simulink model "OdeSimSpring2"  (R2013a)
settings: Solver=ode15s  StartTime=0.0  StopTime=T  MaxStep=1e-3  RelTol=1e-3
InitFcn:
  | m=.015;
  | K=1000;
  | L0=.08;
  | f=1;
  | T=1/f;
  | L0_Ode=.1;
  | D_L0_Ode=.01;
  | R=.016;
  | 
  | % Constant Velocity
  | a1=(3/2*pi)/T;
  | 
  | % constant acceleration
  | a2=2*(3/2*pi)/((T^2));
  | 
  | % sin
  | a3=-(3/4*pi);
  | b3=pi/T;
  | c3=pi/2;
  | d3=-a3;
libraries: simulink x1
settings Model: Creator=root  LastModifiedBy=root

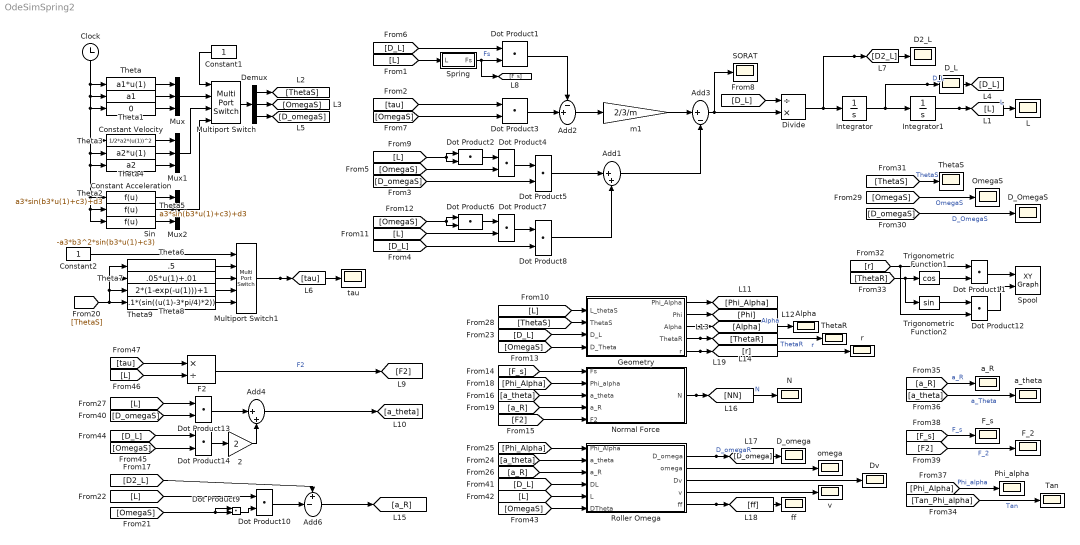
== system OdeSimSpring2 ==
  2 : Gain  Gain=2
  Add1 : Sum  Inputs=|++
  Add2 : Sum  Inputs=-+|
  Add3 : Sum  Inputs=|+-
  Add4 : Sum  Inputs=|++
  Add6 : Sum  Inputs=+-|
  Alpha : Scope
  Clock : Clock
  Constant Acceleration : Fcn  Expr=a2
  Constant Velocity : Fcn  Expr=0
  Constant1 : Constant
  Constant2 : Constant
  D2_L : Scope
      settings: SaveName=ScopeData21
  D_L : Scope
      settings: SaveName=ScopeData22
  D_OmegaS : Scope
      settings: SaveName=ScopeData16
  D_omega : Scope
      settings: TimeRange=1  YMin=-99.79943282286136  YMax=104.2652110780353
  Demux : Demux  Outputs=3
  Divide : Product  Inputs=/*
  Dot Product{1..14} (14 alike) : DotProduct  InputSameDT=on  OutDataTypeStr=Inherit: Inherit via internal rule
  Dv : Scope
      settings: TimeRange=1  YMin=-1.967332415830284  YMax=2.10455506696653  SaveName=ScopeData2
  F2 : Product  Inputs=*/
  F_2 : Scope
      settings: SaveName=ScopeData3
  F_s : Scope
      settings: SaveName=ScopeData4
  Geometry : Subsystem
  Integrator : Integrator  InitialCondition=D_L0_Ode
  Integrator1 : Integrator  InitialCondition=L0_Ode
  L : Scope
      settings: SaveName=ScopeData23
  Multiport Switch : MultiPortSwitch
  Multiport Switch1 : MultiPortSwitch  Inputs=4
  Mux : Mux  Inputs=3
  Mux1 : Mux  Inputs=3
  Mux2 : Mux  Inputs=3
  N : Scope
      settings: SaveName=ScopeData5
  Normal Force : Subsystem
  OmegaS : Scope
      settings: SaveName=ScopeData18
  Phi_alpha : Scope
      settings: SaveName=ScopeData8
  Roller Omega : Subsystem
  SORAT : Scope
      settings: SaveName=ScopeData15
  Sin : Fcn  Expr=-a3*b3^2*sin(b3*u(1)+c3)
  Spool : simulink/Sinks/XY Graph  xmin=-.3  xmax=.3  ymin=-.3  ymax=.3  st=-1
  Spring : Subsystem
  Tan : Scope
      settings: SaveName=ScopeData9
  Theta : Fcn  Expr=a1*u(1)
  Theta1 : Fcn  Expr=a1
  Theta2 : Fcn  Expr=a3*sin(b3*u(1)+c3)+d3
  Theta3 : Fcn  Expr=1/2*a2*(u(1))^2
  Theta4 : Fcn  Expr=a2*u(1)
  Theta5 : Fcn  Expr=a3*sin(b3*u(1)+c3)+d3
  Theta6 : Fcn  Expr=.5
  Theta7 : Fcn  Expr=.05*u(1)+.01
  Theta8 : Fcn  Expr=2*(1-exp(-u(1)))+1
  Theta9 : Fcn  Expr=.1*(sin((u(1)-3*pi/4)*2))
  ThetaR : Scope
      settings: SaveName=ScopeData10
  ThetaS : Scope
      settings: SaveName=ScopeData19
  Trigonometric Function1 : Trigonometry  Operator=cos
  Trigonometric Function2 : Trigonometry
  a_R : Scope
      settings: SaveName=ScopeData6
  a_theta : Scope
      settings: SaveName=ScopeData7
  ff : Scope
      settings: TimeRange=1  YMin=-0.01982572417882734  YMax=0.01972510148135379  SaveName=ScopeData11
  m1 : Gain  Gain=2/3/m
  omega : Scope
      settings: TimeRange=1  YMin=0  YMax=20  SaveName=ScopeData12
  r : Scope
      settings: SaveName=ScopeData13
  tau : Scope
      settings: SaveName=ScopeData20
  v : Scope
      settings: TimeRange=1  YMin=0.4  YMax=0.8  SaveName=ScopeData14
  wires:
  Integrator1/1 -> L/1, [L]  "L"
  Spring/1(Fs) -> [F_s], Dot Product1/2  "Fs"
  Add1/1 -> Add3/2
  Dot Product1/1 -> Add2/1
  Add2/1 -> m1/1
  Integrator/1 -> Integrator1/1, [D_L], D_L/1  "D_L"
  [L] -> Spring/1(L)
  [D_L] -> Dot Product1/1
  [tau] -> Dot Product3/1
  [OmegaS] -> Dot Product3/2
  Dot Product3/1 -> Add2/2
  [L] -> Dot Product2/1, Dot Product2/2
  Dot Product2/1 -> Dot Product4/1
  [OmegaS] -> Dot Product4/2
  [D_omegaS] -> Dot Product5/2
  Dot Product4/1 -> Dot Product5/1
  [OmegaS] -> Dot Product6/2, Dot Product6/1
  Dot Product6/1 -> Dot Product7/1
  [L] -> Dot Product7/2
  [D_L] -> Dot Product8/2
  Dot Product7/1 -> Dot Product8/1
  Dot Product5/1 -> Add1/1
  Dot Product8/1 -> Add1/2
  m1/1 -> Add3/1
  Add3/1 -> Divide/2, SORAT/1
  [D_L] -> Divide/1
  Theta/1 -> Mux/1
  Theta1/1 -> Mux/2
  Constant Velocity/1 -> Mux/3
  Constant1/1 -> Multiport Switch/1
  Mux/1 -> Multiport Switch/2
  Multiport Switch/1 -> Demux/1
  Demux/1 -> [ThetaS]
  Demux/2 -> [OmegaS]
  Demux/3 -> [D_omegaS]
  Theta3/1 -> Mux1/1
  Theta4/1 -> Mux1/2
  Constant Acceleration/1 -> Mux1/3
  Mux1/1 -> Multiport Switch/3
  Clock/1 -> Theta4/1, Sin/1, Theta5/1, Theta2/1, Constant Acceleration/1, Theta3/1, Constant Velocity/1, Theta1/1, Theta/1
  Theta2/1 -> Mux2/1
  Theta5/1 -> Mux2/2
  Sin/1 -> Mux2/3
  Mux2/1 -> Multiport Switch/4
  Theta6/1 -> Multiport Switch1/2
  Theta7/1 -> Multiport Switch1/3
  Theta8/1 -> Multiport Switch1/4
  Theta9/1 -> Multiport Switch1/5
  Constant2/1 -> Multiport Switch1/1
  [ThetaS] -> Theta6/1, Theta7/1, Theta8/1, Theta9/1
  Multiport Switch1/1 -> tau/1, [tau]
  [L] -> Geometry/1(L_thetaS)
  [D2_L] -> Add6/1
  Dot Product10/1 -> Add6/2
  [OmegaS] -> Dot Product9/2, Dot Product9/1
  Dot Product9/1 -> Dot Product10/2
  [L] -> Dot Product10/1
  [F_s] -> Normal Force/1(Fs)
  [a_theta] -> Normal Force/3(a_theta)
  [F2] -> Normal Force/5(F2)
  Normal Force/1(N) -> N/1, [NN]  "N"
  Geometry/1(Phi_Alpha) -> [Phi_Alpha]
  Geometry/3(Alpha) -> Alpha/1, [Alpha]  "Alpha"
  [Phi_Alpha] -> Normal Force/2(Phi_alpha)
  Add6/1 -> [a_R]
  [a_R] -> Normal Force/4(a_R)
  [Phi_Alpha] -> Roller Omega/1(Phi_Alpha)
  [a_theta] -> Roller Omega/2(a_theta)
  [a_R] -> Roller Omega/3(a_R)
  Roller Omega/1(D_omega) -> D_omega/1, [D_omega]  "D_omegaR"
  Roller Omega/5(ff) -> ff/1, [ff]
  [ThetaS] -> Geometry/2(ThetaS)
  Geometry/4(ThetaR) -> ThetaR/1, [ThetaR]  "ThetaR"
  Geometry/5(r) -> [r], r/1  "r"
  [a_R] -> a_R/1  "a_R"
  [a_theta] -> a_theta/1  "a_Theta"
  [F2] -> F_2/1  "F_2"
  [F_s] -> F_s/1  "F_s"
  [Tan_Phi_alpha] -> Tan/1  "Tan"
  [Phi_Alpha] -> Phi_alpha/1  "Phi_alpha"
  Geometry/2(Phi) -> [Phi]
  [D_L] -> Roller Omega/4(DL)
  [L] -> Roller Omega/5(L)
  [OmegaS] -> Roller Omega/6(DTheta)
  Roller Omega/2(omega) -> omega/1
  Roller Omega/3(Dv) -> Dv/1
  Roller Omega/4(v) -> v/1
  [ThetaS] -> ThetaS/1  "ThetaS"
  [OmegaS] -> OmegaS/1  "OmegaS"
  [D_omegaS] -> D_OmegaS/1  "D_OmegaS"
  [ThetaR] -> Trigonometric Function2/1, Trigonometric Function1/1
  [r] -> Dot Product12/2, Dot Product11/1
  Trigonometric Function1/1 -> Dot Product11/2
  Trigonometric Function2/1 -> Dot Product12/1
  Dot Product11/1 -> Spool/1
  Dot Product12/1 -> Spool/2
  Divide/1 -> D2_L/1, [D2_L], Integrator/1
  [D_L] -> Geometry/3(D_L)
  [OmegaS] -> Geometry/4(D_Theta)
  [L] -> Dot Product13/1
  [D_omegaS] -> Dot Product13/2
  [OmegaS] -> Dot Product14/2
  [D_L] -> Dot Product14/1
  Dot Product14/1 -> 2/1
  Dot Product13/1 -> Add4/1
  2/1 -> Add4/2
  Add4/1 -> [a_theta]
  [tau] -> F2/1
  [L] -> F2/2
  F2/1 -> [F2]  "F2"

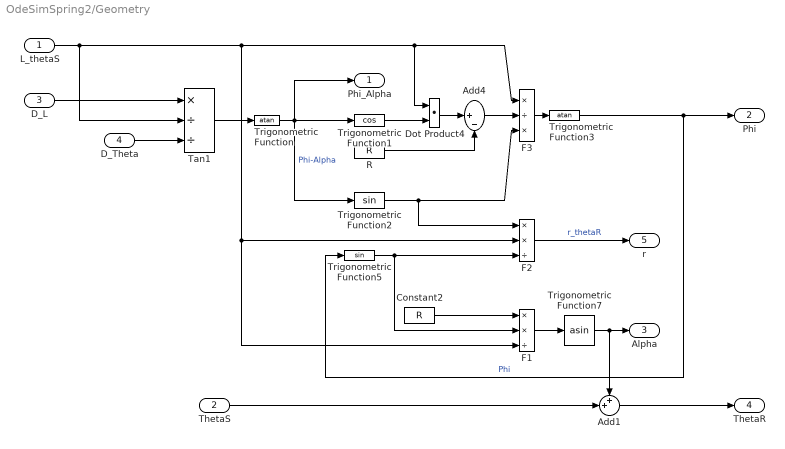
== system OdeSimSpring2/Geometry ==
  L_thetaS : Inport
  ThetaS : Inport  Port=2
  D_L : Inport  Port=3
  D_Theta : Inport  Port=4
  Add1 : Sum  Inputs=++|
  Add4 : Sum  Inputs=|+-
  Constant2 : Constant  Value=R
  Dot Product4 : DotProduct  InputSameDT=on  OutDataTypeStr=Inherit: Inherit via internal rule
  F1 : Product  Inputs=**/
  F2 : Product  Inputs=**/
  F3 : Product  Inputs=*/*
  R : Constant  Value=R
  Tan1 : Product  Inputs=*//
  Trigonometric Function : Trigonometry  Operator=atan
  Trigonometric Function1 : Trigonometry  Operator=cos
  Trigonometric Function2 : Trigonometry
  Trigonometric Function3 : Trigonometry  Operator=atan
  Trigonometric Function5 : Trigonometry
  Trigonometric Function7 : Trigonometry  Operator=asin
  Phi_Alpha : Outport
  Phi : Outport  Port=2
  Alpha : Outport  Port=3
  ThetaR : Outport  Port=4
  r : Outport  Port=5
  wires:
  Tan1/1 -> Trigonometric Function/1
  R/1 -> Add4/2
  Trigonometric Function/1 -> Trigonometric Function2/1, Trigonometric Function1/1, Phi_Alpha/1  "Phi-Alpha"
  Dot Product4/1 -> Add4/1
  Trigonometric Function3/1 -> Trigonometric Function5/1, Phi/1  "Phi"
  F3/1 -> Trigonometric Function3/1
  Trigonometric Function1/1 -> Dot Product4/2
  F2/1 -> r/1  "r_thetaR"
  Constant2/1 -> F1/1
  Trigonometric Function5/1 -> F1/2, F2/3
  F1/1 -> Trigonometric Function7/1
  Trigonometric Function7/1 -> Alpha/1, Add1/1
  Add4/1 -> F3/2
  Trigonometric Function2/1 -> F2/1, F3/3
  ThetaS/1 -> Add1/2
  Add1/1 -> ThetaR/1
  L_thetaS/1 -> Tan1/2, F3/1, Dot Product4/1, F1/3, F2/2
  D_L/1 -> Tan1/1
  D_Theta/1 -> Tan1/3

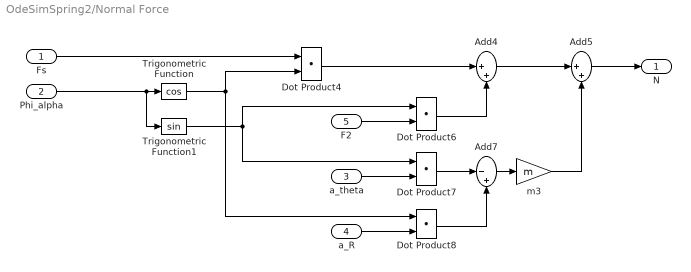
== system OdeSimSpring2/Normal Force ==
  Fs : Inport
  Phi_alpha : Inport  Port=2
  a_theta : Inport  Port=3
  a_R : Inport  Port=4
  F2 : Inport  Port=5
  Add4 : Sum  Inputs=|++
  Add5 : Sum  Inputs=|++
  Add7 : Sum  Inputs=|-+
  Dot Product{4,6..8} (4 alike) : DotProduct  InputSameDT=on  OutDataTypeStr=Inherit: Inherit via internal rule
  Trigonometric Function : Trigonometry  Operator=cos
  Trigonometric Function1 : Trigonometry
  m3 : Gain  Gain=m
  N : Outport
  wires:
  Dot Product6/1 -> Add4/2
  Dot Product8/1 -> Add7/2
  Trigonometric Function/1 -> Dot Product8/1, Dot Product4/2
  m3/1 -> Add5/2
  a_R/1 -> Dot Product8/2
  Add4/1 -> Add5/1
  Dot Product4/1 -> Add4/1
  Dot Product7/1 -> Add7/1
  Add5/1 -> N/1
  Add7/1 -> m3/1
  Phi_alpha/1 -> Trigonometric Function/1, Trigonometric Function1/1
  a_theta/1 -> Dot Product7/2
  Trigonometric Function1/1 -> Dot Product7/1, Dot Product6/1
  F2/1 -> Dot Product6/2
  Fs/1 -> Dot Product4/1

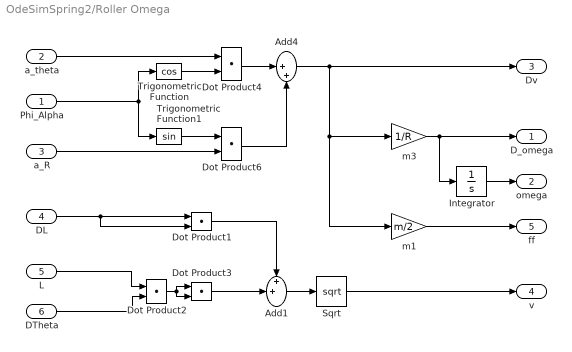
== system OdeSimSpring2/Roller Omega ==
  Phi_Alpha : Inport
  a_theta : Inport  Port=2
  a_R : Inport  Port=3
  DL : Inport  Port=4
  L : Inport  Port=5
  DTheta : Inport  Port=6
  Add1 : Sum  Inputs=++|
  Add4 : Sum  Inputs=|++
  Dot Product{1..4,6} (5 alike) : DotProduct  InputSameDT=on  OutDataTypeStr=Inherit: Inherit via internal rule
  Integrator : Integrator
  Sqrt : Sqrt  SaturateOnIntegerOverflow=on
  Trigonometric Function : Trigonometry  Operator=cos
  Trigonometric Function1 : Trigonometry
  m1 : Gain  Gain=m/2
  m3 : Gain  Gain=1/R
  D_omega : Outport
  omega : Outport  Port=2
  Dv : Outport  Port=3
  v : Outport  Port=4
  ff : Outport  Port=5
  wires:
  Dot Product6/1 -> Add4/2
  m3/1 -> Integrator/1, D_omega/1
  Add4/1 -> Dv/1, m1/1, m3/1
  Trigonometric Function1/1 -> Dot Product6/1
  Phi_Alpha/1 -> Trigonometric Function/1, Trigonometric Function1/1
  a_R/1 -> Dot Product6/2
  Dot Product4/1 -> Add4/1
  a_theta/1 -> Dot Product4/1
  Trigonometric Function/1 -> Dot Product4/2
  m1/1 -> ff/1
  DL/1 -> Dot Product1/2, Dot Product1/1
  L/1 -> Dot Product2/1
  DTheta/1 -> Dot Product2/2
  Dot Product2/1 -> Dot Product3/1, Dot Product3/2
  Dot Product1/1 -> Add1/1
  Dot Product3/1 -> Add1/2
  Add1/1 -> Sqrt/1
  Sqrt/1 -> v/1
  Integrator/1 -> omega/1

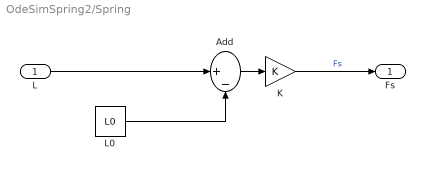
== system OdeSimSpring2/Spring ==
  L : Inport
  Add : Sum  Inputs=|+-
  K : Gain  Gain=K
  L0 : Constant  Value=L0
  Fs : Outport
  wires:
  K/1 -> Fs/1  "Fs"
  Add/1 -> K/1
  L/1 -> Add/1
  L0/1 -> Add/2
